simulink model "verify_Mix_T_Mdot_mdl"  (R2018b)
settings: Solver=VariableStepDiscrete  StartTime=0.0  StopTime=10.0  MaxStep=0.1  RelTol=1e-3  EnableMultiTasking=on
libraries: carnot x3, simulink x2
settings Model: Creator=drhf  LastModifiedBy=drhf
settings DataIOCC: LimitDataPoints=on  SaveFormat=Array
settings OptimizationCC: ExpressionDepthLimit=2147483647  LifeSpan=inf
settings DebuggingCC: UnderspecifiedInitializationDetection=Classic  MergeDetectMultiDrivingBlocksExec=none  SolverPrmCheckMsg=warning  StateNameClashWarn=warning  SFUnexpectedBacktrackingDiag=warning  SFNoUnconditionalDefaultTransitionDiag=warning  SFExecutionAtInitializationDiag=none
settings HardwareCC: ProdBitPerPointer=32  ProdBitPerSizeT=32  ProdBitPerPtrDiffT=32  ProdLargestAtomicFloat=None  ProdIntDivRoundTo=Undefined  ProdEndianess=Unspecified  ProdWordSize=32  ProdHWDeviceType=32-bit Generic
settings ModelReferenceCC: PropagateSignalLabelsOutOfModel=off
settings SFSimCC: SimUseLocalCustomCode=off
settings RTWCC: RTWUseLocalCustomCode=off
settings CodeAppCC: StateflowObjectComments=on
settings GRTTargetCC: TargetLangStandard=C89/C90 (ANSI)  GeneratePreprocessorConditionals=Disable all  CombineOutputUpdateFcns=off  GRTInterface=on
settings ConfigComp: CovMetricSettings=dw  CovHtmlReporting=on  CovSaveCumulativeToWorkspaceVar=on  CovSaveSingleToWorkspaceVar=on  CovExternalEMLEnable=off

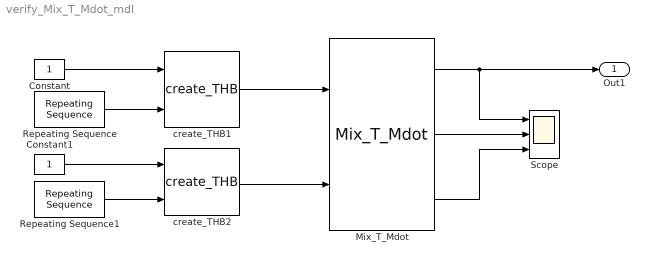
== system verify_Mix_T_Mdot_mdl ==
  Constant : Constant
  Constant1 : Constant
  Mix_T_Mdot : carnot/Basic/Hydraulics/Mix_T_Mdot  mixcalc=Enthalpy balance
  Repeating Sequence : simulink/Sources/Repeating Sequence  rep_seq_t=[0 5 10]  rep_seq_y=[10 50 10]
  Repeating Sequence1 : simulink/Sources/Repeating Sequence  rep_seq_t=[0 5 10]  rep_seq_y=[50 10 50]
  Scope : Scope  NumInputPorts=3
  create_THB1 : carnot/Source/Simple/create_THB  p=1e5  fluid=Air  mix=0.005  mix2=0  mix3=0  dia=0.02  hgt=0  mID=No Pressure Drop
  create_THB2 : carnot/Source/Simple/create_THB  p=1e5  fluid=Air  mix=0.005  mix2=0  mix3=0  dia=0.02  hgt=0  mID=No Pressure Drop
  Out1 : Outport
  wires:
  create_THB1/1 -> Mix_T_Mdot/1
  create_THB2/1 -> Mix_T_Mdot/2
  Constant/1 -> create_THB1/1
  Constant1/1 -> create_THB2/1
  Repeating Sequence/1 -> create_THB1/2
  Repeating Sequence1/1 -> create_THB2/2
  Mix_T_Mdot/1 -> Scope/1, Out1/1
  Mix_T_Mdot/2 -> Scope/2
  Mix_T_Mdot/3 -> Scope/3
